simulink model "pole_cart_dynamics_version_one"  (R2023b)
settings: Solver=FixedStepAuto  StartTime=0  StopTime=20  FixedStep=0.02  MaxStep=0.02  RelTol=1e-3  AbsTol=1e-6
PreLoadFcn:
  | cartpole1
libraries: fuzblock x1
CloseFcn:
  | set(groot,'ShowHiddenHandles','on');
  | c = get(groot,'Children');
  | close(c);
  | clear c;
  | set(groot,'ShowHiddenHandles','off');
Description:
  | Inverted Pendulum with Animation
  | 
  | This example shows how to model an inverted pendulum.  The animation is created using MATLAB(R) Handle Graphics(R).  The animation block is a masked
  | S-function.  For more information, use the context menu to look under the Animation block's mask
  | and open the S-function for editing.
settings Model: Creator=The MathWorks, Inc.  LastModifiedBy=rakshan
settings SolverCC: AutoScaleAbsTol=off  AlgebraicLoopSolver=TrustRegion
settings DataIOCC: ExternalInput=[]  InitialState=[]  SaveFormat=Array  SaveOutput=off  SaveTime=off
settings OptimizationCC: BlockReduction=off  BooleanDataType=off  ReuseModelBlockBuffer=off  ExpressionDepthLimit=2147483647  InitFltsAndDblsToZero=on  LifeSpan=inf
settings DebuggingCC: SaveWithParameterizedLinksMsg=none  UnderspecifiedInitializationDetection=Classic  MergeDetectMultiDrivingBlocksExec=none  SignalResolutionControl=TryResolveAllWithWarning  MultiTaskDSMMsg=warning  MultiTaskCondExecSysMsg=none  SigSpecEnsureSampleTimeMsg=none  FcnCallInpInsideContextMsg=warning  UnconnectedInputMsg=warning  UnconnectedOutputMsg=warning  UnconnectedLineMsg=warning  StateNameClashWarn=warning  SubsystemReferenceDiagnosticForUnitTest=warning  SFUnexpectedBacktrackingDiag=warning  SFNoUnconditionalDefaultTransitionDiag=warning  SFExecutionAtInitializationDiag=none  ArithmeticOperatorsInVariantConditions=warning
settings HardwareCC: ProdBitPerPointer=32  ProdBitPerSizeT=32  ProdBitPerPtrDiffT=32  ProdLargestAtomicFloat=None  ProdIntDivRoundTo=Undefined  ProdEndianess=Unspecified  ProdWordSize=32  ProdHWDeviceType=32-bit Generic  TargetUnknown=on
settings ModelReferenceCC: EnableRefExpFcnMdlSchedulingChecks=on  PropagateSignalLabelsOutOfModel=off
settings SFSimCC: SimUseLocalCustomCode=off  CustomCodeUndefinedFunction=UseInterfaceOnly
settings RTWCC: RTWUseLocalCustomCode=off
settings CodeAppCC: StateflowObjectComments=on
settings GRTTargetCC: TargetFcnLib=ansi_tfl_tmw.mat  TargetLangStandard=C89/C90 (ANSI)  CombineOutputUpdateFcns=off  GRTInterface=on
settings ConfigComp: CovMetricSettings=dw  CovSaveCumulativeToWorkspaceVar=on  CovSaveSingleToWorkspaceVar=on  CovExternalEMLEnable=off

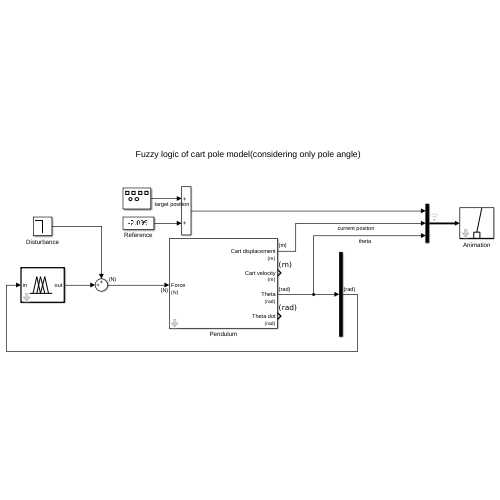
[thumbnail: Simulink's stored preview of the top-level diagram]
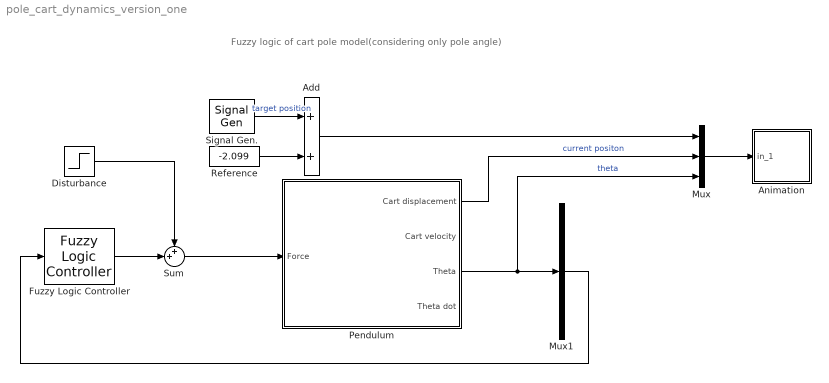
== system pole_cart_dynamics_version_one ==
  note: Fuzzy logic of cart pole model(considering only pole angle)
  Add : Sum
  Animation : Subsystem  mask(Pendulum plot){RefBlock=Reference}
      mask prompts: RefBlock "DC reference signal block name:"
      mask help: Pendulum plot
      mask Help: Pendulum animation function using Handle graphics.
      mask Display: plot([-10 10],[0 0],[-2 -2 2 2],[0 1 1 0],[0 3],[1 5])
  Disturbance : Step  Before=1  After=0  SampleTime=0
  Fuzzy Logic Controller : fuzblock/Fuzzy Logic  Controller  FIS=cartpole1FIS  OutputSampleNumber=101  DataType=double  FuzzifiedInputs=off  RuleFiringStrengths=off  RuleOutputs=off  AggregatedOutputs=off  SimulateUsing=Interpreted execution  OutOfRangeInputValueMessage=warning  NoRuleFiredMessage=warning  EmptyOutputFuzzySetMessage=warning
  Mux : Mux  Inputs=3
  Mux1 : Mux  Inputs=1
  Pendulum : Subsystem  mask(Inverted Pendulum Dynamics){Mcart=0.455, m=0.21, l=0.61/2, g=9.8}
      mask prompts: Mcart "Mass of cart (kg):"; m "Mass of pendulum (kg):"; l "Distance to pendulum center of mass (m):"; g "Acceleration of gravity (m/s^2):"
      mask help: Masked subsystem containing nonlinear dynamics of inverted pendulum on a cart.
      mask Help: Nonlinear dynamics of inverted pendulum on cart.
  Reference : Constant  Value=-2.099
  Signal Gen. : SignalGenerator  WaveForm=square  Amplitude=0  Frequency=0.0400000  Units=rad/sec
  Sum : Sum  Inputs=++|
  wires:
  Mux/1 -> Animation/1(in_1)
  Pendulum/3(Theta) -> Mux/3, Mux1/1  "theta"
  Pendulum/1(Cart displacement) -> Mux/2  "current positon"
  Signal Gen./1 -> Add/1  "target position"
  Reference/1 -> Add/2
  Add/1 -> Mux/1
  Sum/1 -> Pendulum/1(Force)
  Fuzzy Logic Controller/1 -> Sum/2
  Disturbance/1 -> Sum/1
  Mux1/1 -> Fuzzy Logic Controller/1

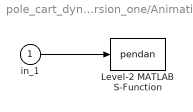
== system pole_cart_dynamics_version_one/Animation ==
  in_1 : Inport
  Level-2 MATLAB S-Function : M-S-Function  FunctionName=pendan  Parameters=RefBlock
  wires:
  in_1/1 -> Level-2 MATLAB S-Function/1

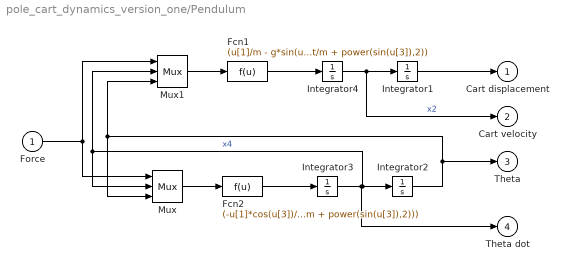
== system pole_cart_dynamics_version_one/Pendulum ==
  Force : Inport  Unit=N
  Fcn1 : Fcn  Expr=(u[1]/m - g*sin(u[3])*cos(u[3]) + l*power(u[2],2)*sin(u[3]))/(Mcart/m + power(sin(u[3]),2))
  Fcn2 : Fcn  Expr=(-u[1]*cos(u[3])/m + (Mcart+m)*g*sin(u[3])/m - l*power(u[2],2)*sin(u[3])*cos(u[3]))/(l*(Mcart/m + power(sin(u[3]),2)))
  Integrator{1..4} (4 alike) : Integrator
  Mux : Mux  Inputs=3
  Mux1 : Mux  Inputs=3
  Cart displacement : Outport  Unit=m  InitialOutput=0  VectorParamsAs1DForOutWhenUnconnected=off
  Cart velocity : Outport  Port=2  Unit=m  InitialOutput=0  VectorParamsAs1DForOutWhenUnconnected=off
  Theta : Outport  Port=3  Unit=rad  InitialOutput=0  VectorParamsAs1DForOutWhenUnconnected=off
  Theta dot : Outport  Port=4  Unit=rad  InitialOutput=0  VectorParamsAs1DForOutWhenUnconnected=off
  wires:
  Integrator1/1 -> Cart displacement/1
  Fcn2/1 -> Integrator3/1
  Mux/1 -> Fcn2/1
  Mux1/1 -> Fcn1/1
  Fcn1/1 -> Integrator4/1
  Integrator4/1 -> Cart velocity/1, Integrator1/1  "x2"
  Force/1 -> Mux1/1, Mux/1
  Integrator3/1 -> Theta dot/1, Integrator2/1, Mux1/2, Mux/2  "x4"
  Integrator2/1 -> Mux1/3, Mux/3, Theta/1
